simulink model "sampleModel115"  (R2021b)
settings: Solver=VariableStepAuto  StartTime=0.0  StopTime=10.0  RelTol=1e-3
undefined symbols (not defined in the file or in its folder): DiscIntNeverNeededParam
libraries: simulink x4, slpidlib x2
settings Model: Creator=user  LastModifiedBy=user

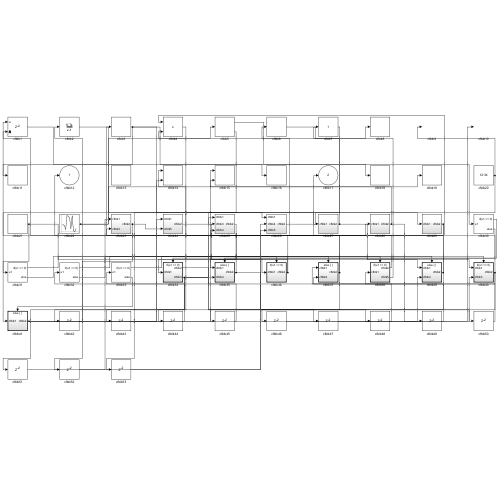
[thumbnail: Simulink's stored preview of the top-level diagram]
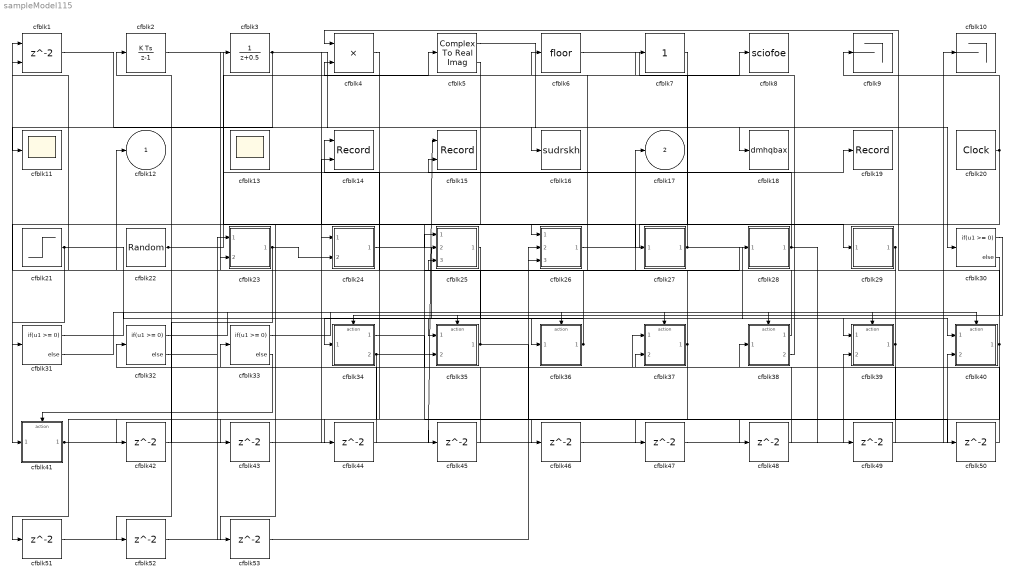
== system sampleModel115 ==
  cfblk1 : Delay  ShowEnablePort=on  SampleTime=1
      settings: InputPortMap=u0,e6
  cfblk10 : Terminator
  cfblk11 : Scope
  cfblk13 : Scope
      settings: Floating=on
  cfblk14 : Record  FileSettingsInternal="{\"entries\":[{\"content\":{\"excelSettings\":{\"content\":{},\"type\":\"Streamout.ExcelSettings\"}},\"type\":\"Streamout.FileSettingStorage\",\"uuid\":\"b1ceb9cc-7e03-40a6-99d7-b30e3dfb90d7\"}],\"packageUris\":[\"http://schema.mathworks.com/mf0/streamout_blocks/R2020a\"],\"version\":\"1.0\"}"  Layout=[1 1]  SignalsInternal="{\"entries\":[{\"content\":{\"signals\":[{\"content\":{\"blockPath\":[\"sampleModel115/cfblk14\"],\"channel\":[],\"dimensions\":[1],\"domain\":\"sampleModel115/cfblk14\",\"lineColor\":\"#a2142f\",\"plots\":[1],\"port\":1,\"sid\":[\"\"],\"signalID\":4053,\"signalName\":\"cfblk36\"},\"type\":\"RecordBlkView.Signal\",\"uuid\":\"947220fe-0bb9-4a12-b0be-18da4abc70e8\"},{\"content\":{\"blockPath\":[\"sampleModel115/cfblk14\"],\"channel\":[],\"dimensions\":[1],\"domain\":\"sampleModel115/cfblk14\",\"lineColor\":\"#139fff\",\"plots\":[1],\"port\":2,\"sid\":[\"\"],\"signalID\":4057,\"signalName\":\"cfblk41\"},\"type\":\"RecordBlkView.Signal\",\"uuid\":\"8ca9a1bb-19d5-482f-8e05-41f11873065c\"}]},\"type\":\"RecordBlkView.InputSignals\",\"uuid\":\"13a21eec-39b3-41d5-bfac-9f26ae1d7b34\"}],\"packageUris\":[\"http://schema.mathworks.com/mf0/streamout_blocks/R2020a\"],\"version\":\"1.0\"}"  VisualizationBindings="{\"xyplotplugin\":{\"info\":[{\"series\":[{\"bindingParametersList\":[{\"parameter\":\"X-Axis\",\"signalID\":4053,\"signalName\":\"cfblk36\"},{\"parameter\":\"Y-Axis\",\"signalID\":4057,\"signalName\":\"cfblk41\"}],\"seriesID\":55927}],\"subplotID\":1}]}}"  CompatibilityTag=XY
  cfblk15 : Record  FileSettingsInternal="{\"entries\":[{\"content\":{\"excelSettings\":{\"content\":{},\"type\":\"Streamout.ExcelSettings\"}},\"type\":\"Streamout.FileSettingStorage\",\"uuid\":\"98b4cf14-7218-4872-a4ba-8d7d1830e3d3\"}],\"packageUris\":[\"http://schema.mathworks.com/mf0/streamout_blocks/R2020a\"],\"version\":\"1.0\"}"  Layout=[1 1]  SignalsInternal="{\"entries\":[{\"content\":{\"signals\":[{\"content\":{\"blockPath\":[\"sampleModel115/cfblk15\"],\"channel\":[],\"dimensions\":[1],\"domain\":\"sampleModel115/cfblk15\",\"lineColor\":\"#a2142f\",\"plots\":[1],\"port\":1,\"sid\":[\"\"],\"signalID\":4061,\"signalName\":\"cfblk41\"},\"type\":\"RecordBlkView.Signal\",\"uuid\":\"48149283-0b4a-4ff8-890c-8be74494f9ea\"},{\"content\":{\"blockPath\":[\"sampleModel115/cfblk15\"],\"channel\":[],\"dimensions\":[1],\"domain\":\"sampleModel115/cfblk15\",\"lineColor\":\"#139fff\",\"plots\":[1],\"port\":2,\"sid\":[\"\"],\"signalID\":4065,\"signalName\":\"cfblk28\"},\"type\":\"RecordBlkView.Signal\",\"uuid\":\"1207e1b5-9b3d-40f8-9197-40b30a57e16f\"}]},\"type\":\"RecordBlkView.InputSignals\",\"uuid\":\"f4e16f90-73cc-457e-a6ee-f5fba29a4091\"}],\"packageUris\":[\"http://schema.mathworks.com/mf0/streamout_blocks/R2020a\"],\"version\":\"1.0\"}"  VisualizationBindings="{\"xyplotplugin\":{\"info\":[{\"series\":[{\"bindingParametersList\":[{\"parameter\":\"X-Axis\",\"signalID\":4061,\"signalName\":\"cfblk41\"},{\"parameter\":\"Y-Axis\",\"signalID\":4065,\"signalName\":\"cfblk28\"}],\"seriesID\":28598}],\"subplotID\":1}]}}"  CompatibilityTag=XY
  cfblk16 : ToWorkspace  VariableName=sudrskh  SaveFormat=Timeseries  SampleTime=-1
  cfblk18 : ToWorkspace  VariableName=dmhqbax  SaveFormat=Timeseries  SampleTime=-1
  cfblk19 : Record  FileSettingsInternal="{\"entries\":[{\"content\":{\"excelSettings\":{\"content\":{},\"type\":\"Streamout.ExcelSettings\"}},\"type\":\"Streamout.FileSettingStorage\",\"uuid\":\"cad0cdc5-0fe9-49e7-8a7a-dd39cebd2482\"}],\"packageUris\":[\"http://schema.mathworks.com/mf0/streamout_blocks/R2020a\"],\"version\":\"1.0\"}"  SignalsInternal="{\"entries\":[{\"content\":{\"signals\":[{\"content\":{\"blockPath\":[\"sampleModel115/cfblk19\"],\"channel\":[],\"dimensions\":[1],\"domain\":\"sampleModel115/cfblk19\",\"lineColor\":\"#d95319\",\"plots\":[1],\"port\":1,\"sid\":[\"\"],\"signalID\":4069,\"signalName\":\"cfblk22\"},\"type\":\"RecordBlkView.Signal\",\"uuid\":\"e627ca45-b87b-4f08-af19-0e4785aecbb7\"}]},\"type\":\"RecordBlkView.InputSignals\",\"uuid\":\"f235e641-5202-4a38-b892-f540294f6c47\"}],\"packageUris\":[\"http://schema.mathworks.com/mf0/streamout_blocks/R2020a\"],\"version\":\"1.0\"}"  VisualizationBindings="{\"sparklinesplugin\":{\"info\":[{\"bindingParametersList\":[],\"subplotID\":1}]}}"
  cfblk2 : DiscreteIntegrator  ICPrevOutput=DiscIntNeverNeededParam  ICPrevScaledInput=DiscIntNeverNeededParam
  cfblk20 : DigitalClock
  cfblk21 : Step  Time=[16.000000]  Before=[-107082885.337694]  After=[-216518547.017650]  SampleTime=0
  cfblk22 : RandomNumber  Mean=[-52247.991135]  Variance=[91177.306892]  Seed=[709185033.000000]  SampleTime=0.1
  cfblk23 : Subsystem
  cfblk24 : Subsystem
  cfblk25 : Subsystem
  cfblk26 : Subsystem
  cfblk27 : Subsystem
  cfblk28 : Subsystem
  cfblk29 : Subsystem
  cfblk3 : DiscreteTransferFcn  SampleTime=1
  cfblk{30..33} (4 alike) : If  IfExpression=u1 >= 0  SampleTime=1
  cfblk34 : Subsystem  TreatAsAtomicUnit=on
  cfblk35 : Subsystem  TreatAsAtomicUnit=on
  cfblk36 : Subsystem  TreatAsAtomicUnit=on
  cfblk37 : Subsystem  TreatAsAtomicUnit=on
  cfblk38 : Subsystem  TreatAsAtomicUnit=on
  cfblk39 : Subsystem  TreatAsAtomicUnit=on
  cfblk4 : Product  Inputs=**
  cfblk40 : Subsystem  TreatAsAtomicUnit=on
  cfblk41 : Subsystem  TreatAsAtomicUnit=on
  cfblk{42..53} (12 alike) : Delay  SampleTime=1
  cfblk5 : ComplexToRealImag
  cfblk6 : Rounding
  cfblk7 : simulink/Math Operations/Slider Gain  gain=1  low=0  high=2
  cfblk8 : ToWorkspace  VariableName=sciofoe  SaveFormat=Timeseries  SampleTime=-1
  cfblk9 : Terminator
  cfblk12 : Outport
  cfblk17 : Outport  Port=2
  wires:
  cfblk3/1 -> cfblk16/1, cfblk11/1, cfblk27/1(cfblk1)
  cfblk23/1(cfblk2) -> cfblk24/2(cfblk5), cfblk42/1
  cfblk26/1(cfblk2) -> cfblk29/1(cfblk1)
  cfblk40/1(cfblk2) -> cfblk4/1, cfblk37/2(cfblk4), cfblk45/1
  cfblk29/1(cfblk2) -> cfblk1/1, cfblk23/2(cfblk3)
  cfblk24/1(cfblk2) -> cfblk39/1(cfblk1)
  cfblk25/1(cfblk2) -> cfblk34/1(cfblk1)
  cfblk20/1 -> cfblk9/1, cfblk25/2(cfblk3)
  cfblk37/1(cfblk2) -> cfblk17/1, cfblk25/3(cfblk4), cfblk46/1
  cfblk6/1 -> cfblk8/1
  cfblk41/1(cfblk2) -> cfblk15/1, cfblk14/2, cfblk10/1
  cfblk2/1 -> cfblk26/1(cfblk1)
  cfblk22/1 -> cfblk19/1, cfblk5/1
  cfblk36/1(cfblk2) -> cfblk14/1, cfblk35/1(cfblk1)
  cfblk5/1 -> cfblk30/1
  cfblk5/2 -> cfblk41/1(cfblk1)
  cfblk28/1(cfblk2) -> cfblk15/2, cfblk49/1
  cfblk39/1(cfblk2) -> cfblk3/1, cfblk1/2, cfblk53/1
  cfblk21/1 -> cfblk36/1(cfblk1), cfblk31/1
  cfblk34/2(cfblk3) -> cfblk28/1(cfblk1), cfblk35/2(cfblk4), cfblk48/1, cfblk51/1, cfblk52/1
  cfblk38/1(cfblk2) -> cfblk6/1
  cfblk27/1(cfblk2) -> cfblk7/1, cfblk40/1(cfblk1)
  cfblk1/1 -> cfblk18/1
  cfblk35/1(cfblk2) -> cfblk12/1, cfblk50/1
  cfblk38/2(cfblk5) -> cfblk4/2
  cfblk30/1 -> cfblk34/Action
  cfblk30/2 -> cfblk35/Action
  cfblk31/1 -> cfblk36/Action
  cfblk31/2 -> cfblk37/Action
  cfblk32/1 -> cfblk38/Action
  cfblk32/2 -> cfblk39/Action
  cfblk33/1 -> cfblk40/Action
  cfblk33/2 -> cfblk41/Action
  cfblk42/1 -> cfblk2/1
  cfblk7/1 -> cfblk43/1
  cfblk43/1 -> cfblk24/1(cfblk1)
  cfblk4/1 -> cfblk44/1
  cfblk44/1 -> cfblk33/1
  cfblk45/1 -> cfblk32/1
  cfblk46/1 -> cfblk40/2(cfblk3)
  cfblk34/1(cfblk2) -> cfblk47/1
  cfblk47/1 -> cfblk39/2(cfblk4)
  cfblk48/1 -> cfblk38/1(cfblk1)
  cfblk49/1 -> cfblk37/1(cfblk1)
  cfblk50/1 -> cfblk25/1(cfblk1)
  cfblk51/1 -> cfblk23/1(cfblk1)
  cfblk52/1 -> cfblk26/2(cfblk4)
  cfblk53/1 -> cfblk26/3(cfblk5)

== system sampleModel115/cfblk23 ==
  cfblk1 : Inport
  cfblk3 : Inport  Port=2
  cfblk2 : Outport
  wires:
  cfblk1/1 -> cfblk2/1

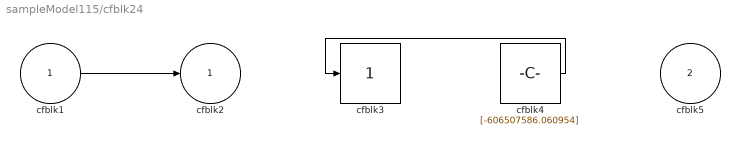
== system sampleModel115/cfblk24 ==
  cfblk1 : Inport
  cfblk5 : Inport  Port=2
  cfblk3 : simulink/Math Operations/Slider Gain  gain=1  low=0  high=2
  cfblk4 : Constant  Value=[-606507586.060954]  SampleTime=1
  cfblk2 : Outport
  wires:
  cfblk1/1 -> cfblk2/1
  cfblk4/1 -> cfblk3/1

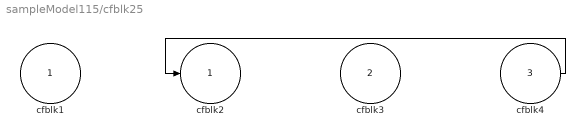
== system sampleModel115/cfblk25 ==
  cfblk1 : Inport
  cfblk3 : Inport  Port=2
  cfblk4 : Inport  Port=3
  cfblk2 : Outport
  wires:
  cfblk4/1 -> cfblk2/1

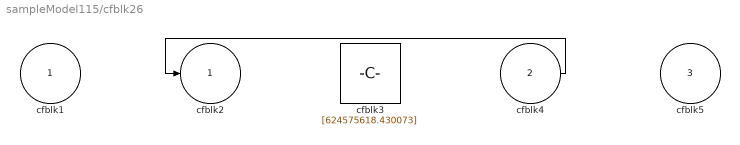
== system sampleModel115/cfblk26 ==
  cfblk1 : Inport
  cfblk4 : Inport  Port=2
  cfblk5 : Inport  Port=3
  cfblk3 : Constant  Value=[624575618.430073]  SampleTime=1
  cfblk2 : Outport
  wires:
  cfblk4/1 -> cfblk2/1

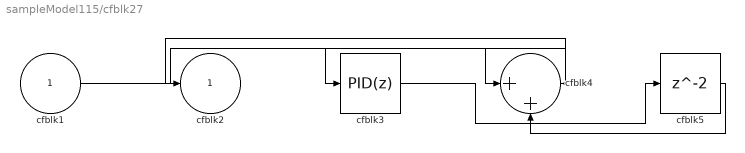
== system sampleModel115/cfblk27 ==
  cfblk1 : Inport
  cfblk3 : slpidlib/PID Controller  Controller=PID  Form=Parallel  TimeDomain=Discrete-time  UseExternalTs=off  SampleTime=1  IntegratorMethod=Forward Euler  FilterMethod=Forward Euler  ControllerParametersSource=internal  P=1  I=1  D=0  UseFilter=on  N=100  TunerSelectOption=Transfer Function Based (PID Tuner App)  InitialConditionSource=internal  InitialConditionForIntegrator=0  InitialConditionForFilter=0  DifferentiatorICPrevScaledInput=0  ExternalReset=none  TrackingMode=off  Kt=1  LimitOutput=off  SatLimitsSource=internal  UpperSaturationLimit=inf  LowerSaturationLimit=-inf  LinearizeAsGain=off  AntiWindupMode=none  Kb=1  POutMin=[]  POutMax=[]  IOutMin=[]  IOutMax=[]  DOutMin=[]  DOutMax=[]  NOutMin=[]  NOutMax=[]  SumOutMin=[]  SumOutMax=[]  SaturationOutMin=[]  SaturationOutMax=[]  PParamMin=[]  PParamMax=[]  IParamMin=[]  IParamMax=[]  DParamMin=[]  DParamMax=[]  NParamMin=[]  NParamMax=[]  KbParamMin=[]  KbParamMax=[]  KtParamMin=[]  KtParamMax=[]  KbOutMin=[]  KbOutMax=[]  KtOutMin=[]  KtOutMax=[]  IntegratorOutMin=[]  IntegratorOutMax=[]  FilterOutMin=[]  FilterOutMax=[]  SumI1OutMin=[]  SumI1OutMax=[]  SumI2OutMin=[]  SumI2OutMax=[]  SumI3OutMin=[]  SumI3OutMax=[]  SumI4OutMin=[]  SumI4OutMax=[]  SumDOutMin=[]  SumDOutMax=[]  DifferentiatorOutMin=[]  DifferentiatorOutMax=[]  FilterDiffOutCoefMin=[]  FilterDiffOutCoefMax=[]  ReciprocalOutMin=[]  ReciprocalOutMax=[]  SumDenOutMin=[]  SumDenOutMax=[]  SumNumOutMin=[]  SumNumOutMax=[]  DivideOutMin=[]  DivideOutMax=[]  UdiffTsProdOutMin=[]  UdiffTsProdOutMax=[]  NTsProdOutMin=[]  NTsProdOutMax=[]  UintegralTsProdOutMin=[]  UintegralTsProdOutMax=[]  UngainTsProdOutMin=[]  UngainTsProdOutMax=[]  IntegratorContinuousStateAttributes=''  IntegratorStateMustResolveToSignalObject=off  IntegratorRTWStateStorageClass=Auto  FilterContinuousStateAttributes=''  FilterStateMustResolveToSignalObject=off  FilterRTWStateStorageClass=Auto  ParallelPVariant=InternalParameters  IdealPVariant=Disabled  IVariant=InternalParameters  DVariant=InternalParameters  IntegratorVariant=Discrete  SatVariant=Disabled  AWVariant=Passthrough  PCopyVariant=Disabled  TRVariant=Disabled  FdbkBlocksVariant=Forward  IdealPFdbkVariant=Disabled  SatFdbkVariant=Disabled  DerivativeFilterVariant=ForwardEulerFilter  NVariant=InternalParameters  NCopyVariant=Disabled  FilterICVariant=InternalICsFilter  IntegratorICVariant=InternalICs  ExternalResetVariant=Disabled  TRSumVariant=Passthrough  SumFdbkVariant=Disabled  SumVariant=Sum_PID  TsampFilterVariant=InternalTs  TsampNgainVariant=Passthrough  TsampIntegralVariant=Passthrough  ExternalSaturationOutDataTypeStr=Inherit: Same as second input
  cfblk4 : Sum  Inputs=|++
  cfblk5 : Delay  SampleTime=1
  cfblk2 : Outport
  wires:
  cfblk1/1 -> cfblk4/1
  cfblk4/1 -> cfblk2/1, cfblk3/1
  cfblk3/1 -> cfblk5/1
  cfblk5/1 -> cfblk4/2

== system sampleModel115/cfblk28 ==
  cfblk1 : Inport
  cfblk3 : simulink/Discrete/Transfer Fcn Real Zero  ZeroZ=0.75  ICPrevInput=0.0  DoSatur=off
      settings: SourceProductBaseCode=SL
  cfblk2 : Outport
  wires:
  cfblk3/1 -> cfblk2/1
  cfblk1/1 -> cfblk3/1

== system sampleModel115/cfblk29 ==
  cfblk1 : Inport
  cfblk3 : MinMax  Function=max
  cfblk2 : Outport
  wires:
  cfblk3/1 -> cfblk2/1
  cfblk1/1 -> cfblk3/1

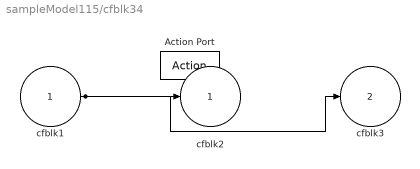
== system sampleModel115/cfblk34 ==
  cfblk1 : Inport
  Action Port : ActionPort  ActionPortLabel=if(u1 >= 0)
  cfblk2 : Outport
  cfblk3 : Outport  Port=2
  wires:
  cfblk1/1 -> cfblk3/1, cfblk2/1

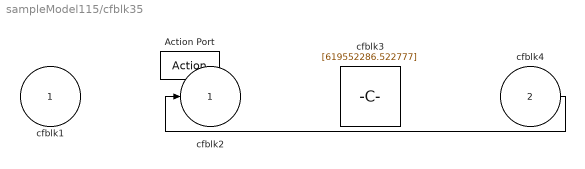
== system sampleModel115/cfblk35 ==
  cfblk1 : Inport
  cfblk4 : Inport  Port=2
  Action Port : ActionPort  ActionPortLabel=else
  cfblk3 : Constant  Value=[619552286.522777]  SampleTime=1
  cfblk2 : Outport
  wires:
  cfblk4/1 -> cfblk2/1

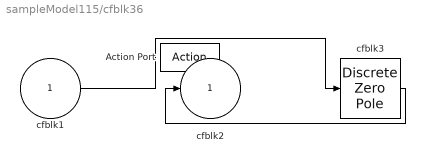
== system sampleModel115/cfblk36 ==
  cfblk1 : Inport
  Action Port : ActionPort  ActionPortLabel=if(u1 >= 0)
  cfblk3 : DiscreteZeroPole  Poles=[0 0.5]  Gain=1  SampleTime=-1
  cfblk2 : Outport
  wires:
  cfblk3/1 -> cfblk2/1
  cfblk1/1 -> cfblk3/1

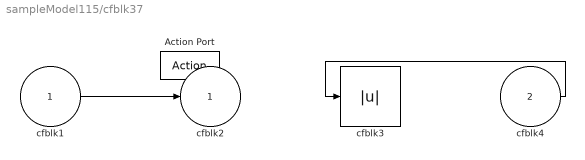
== system sampleModel115/cfblk37 ==
  cfblk1 : Inport
  cfblk4 : Inport  Port=2
  Action Port : ActionPort  ActionPortLabel=else
  cfblk3 : Abs
  cfblk2 : Outport
  wires:
  cfblk1/1 -> cfblk2/1
  cfblk4/1 -> cfblk3/1

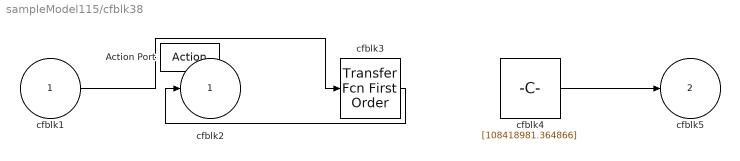
== system sampleModel115/cfblk38 ==
  cfblk1 : Inport
  Action Port : ActionPort  ActionPortLabel=if(u1 >= 0)
  cfblk3 : simulink/Discrete/Transfer Fcn First Order  PoleZ=0.95  ICPrevOutput=0.0  DoSatur=off
  cfblk4 : Constant  Value=[108418981.364866]  SampleTime=1
  cfblk2 : Outport
  cfblk5 : Outport  Port=2
  wires:
  cfblk4/1 -> cfblk5/1
  cfblk3/1 -> cfblk2/1
  cfblk1/1 -> cfblk3/1

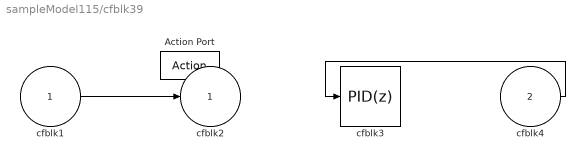
== system sampleModel115/cfblk39 ==
  cfblk1 : Inport
  cfblk4 : Inport  Port=2
  Action Port : ActionPort  ActionPortLabel=else
  cfblk3 : slpidlib/PID Controller  Controller=PID  Form=Parallel  TimeDomain=Discrete-time  UseExternalTs=off  SampleTime=-1  IntegratorMethod=Forward Euler  FilterMethod=Forward Euler  ControllerParametersSource=internal  P=1  I=1  D=0  UseFilter=on  N=100  TunerSelectOption=Transfer Function Based (PID Tuner App)  InitialConditionSource=internal  InitialConditionForIntegrator=0  InitialConditionForFilter=0  DifferentiatorICPrevScaledInput=0  ExternalReset=none  TrackingMode=off  Kt=1  LimitOutput=off  SatLimitsSource=internal  UpperSaturationLimit=inf  LowerSaturationLimit=-inf  LinearizeAsGain=off  AntiWindupMode=none  Kb=1  POutMin=[]  POutMax=[]  IOutMin=[]  IOutMax=[]  DOutMin=[]  DOutMax=[]  NOutMin=[]  NOutMax=[]  SumOutMin=[]  SumOutMax=[]  SaturationOutMin=[]  SaturationOutMax=[]  PParamMin=[]  PParamMax=[]  IParamMin=[]  IParamMax=[]  DParamMin=[]  DParamMax=[]  NParamMin=[]  NParamMax=[]  KbParamMin=[]  KbParamMax=[]  KtParamMin=[]  KtParamMax=[]  KbOutMin=[]  KbOutMax=[]  KtOutMin=[]  KtOutMax=[]  IntegratorOutMin=[]  IntegratorOutMax=[]  FilterOutMin=[]  FilterOutMax=[]  SumI1OutMin=[]  SumI1OutMax=[]  SumI2OutMin=[]  SumI2OutMax=[]  SumI3OutMin=[]  SumI3OutMax=[]  SumI4OutMin=[]  SumI4OutMax=[]  SumDOutMin=[]  SumDOutMax=[]  DifferentiatorOutMin=[]  DifferentiatorOutMax=[]  FilterDiffOutCoefMin=[]  FilterDiffOutCoefMax=[]  ReciprocalOutMin=[]  ReciprocalOutMax=[]  SumDenOutMin=[]  SumDenOutMax=[]  SumNumOutMin=[]  SumNumOutMax=[]  DivideOutMin=[]  DivideOutMax=[]  UdiffTsProdOutMin=[]  UdiffTsProdOutMax=[]  NTsProdOutMin=[]  NTsProdOutMax=[]  UintegralTsProdOutMin=[]  UintegralTsProdOutMax=[]  UngainTsProdOutMin=[]  UngainTsProdOutMax=[]  IntegratorContinuousStateAttributes=''  IntegratorStateMustResolveToSignalObject=off  IntegratorRTWStateStorageClass=Auto  FilterContinuousStateAttributes=''  FilterStateMustResolveToSignalObject=off  FilterRTWStateStorageClass=Auto  ParallelPVariant=InternalParameters  IdealPVariant=Disabled  IVariant=InternalParameters  DVariant=InternalParameters  IntegratorVariant=Discrete  SatVariant=Disabled  AWVariant=Passthrough  PCopyVariant=Disabled  TRVariant=Disabled  FdbkBlocksVariant=Forward  IdealPFdbkVariant=Disabled  SatFdbkVariant=Disabled  DerivativeFilterVariant=ForwardEulerFilter  NVariant=InternalParameters  NCopyVariant=Disabled  FilterICVariant=InternalICsFilter  IntegratorICVariant=InternalICs  ExternalResetVariant=Disabled  TRSumVariant=Passthrough  SumFdbkVariant=Disabled  SumVariant=Sum_PID  TsampFilterVariant=InternalTs  TsampNgainVariant=Passthrough  TsampIntegralVariant=Passthrough  ExternalSaturationOutDataTypeStr=Inherit: Same as second input
  cfblk2 : Outport
  wires:
  cfblk1/1 -> cfblk2/1
  cfblk4/1 -> cfblk3/1

== system sampleModel115/cfblk40 ==
  cfblk1 : Inport
  cfblk3 : Inport  Port=2
  Action Port : ActionPort  ActionPortLabel=if(u1 >= 0)
  cfblk2 : Outport
  wires:
  cfblk1/1 -> cfblk2/1

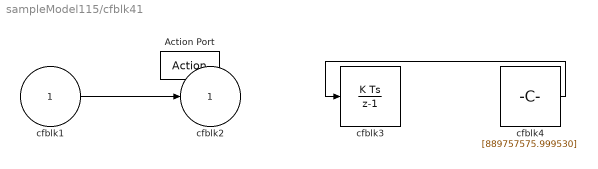
== system sampleModel115/cfblk41 ==
  cfblk1 : Inport
  Action Port : ActionPort  ActionPortLabel=else
  cfblk3 : DiscreteIntegrator  SampleTime=-1  ICPrevOutput=DiscIntNeverNeededParam  ICPrevScaledInput=DiscIntNeverNeededParam
  cfblk4 : Constant  Value=[889757575.999530]  SampleTime=1
  cfblk2 : Outport
  wires:
  cfblk4/1 -> cfblk3/1
  cfblk1/1 -> cfblk2/1
